simulink model "Fuzzy_PID"  (R2022b)
settings: Solver=FixedStepAuto  StartTime=0.0  StopTime=0.1  FixedStep=0.001  RelTol=1e-3
libraries: fuzblock x1
settings Model: Creator=zhouwenjie  LastModifiedBy=zhouwenjie

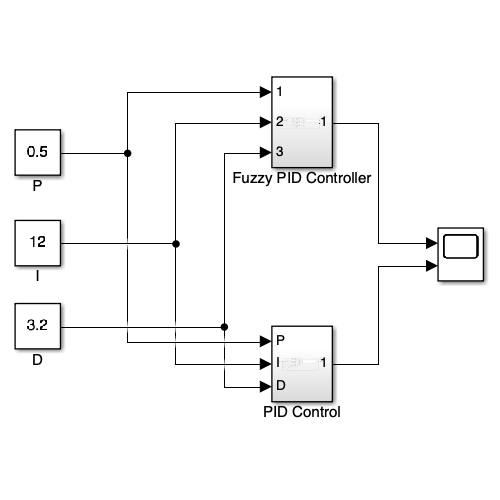
[thumbnail: Simulink's stored preview of the top-level diagram]
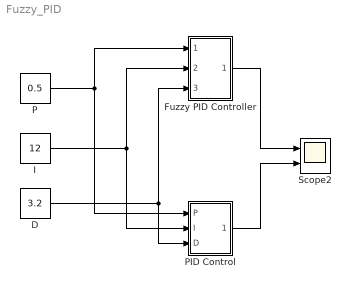
== system Fuzzy_PID ==
  D : Constant  Value=3.2
  Fuzzy PID Controller : Subsystem
  I : Constant  Value=12
  P : Constant  Value=0.5
  PID Control : Subsystem
  Scope2 : Scope  NumInputPorts=2
  wires:
  P/1 -> PID Control/1(P), Fuzzy PID Controller/1(In1)
  I/1 -> PID Control/2(I), Fuzzy PID Controller/2(In2)
  D/1 -> Fuzzy PID Controller/3(In3), PID Control/3(D)
  PID Control/1(Output) -> Scope2/2
  Fuzzy PID Controller/1(Out1) -> Scope2/1

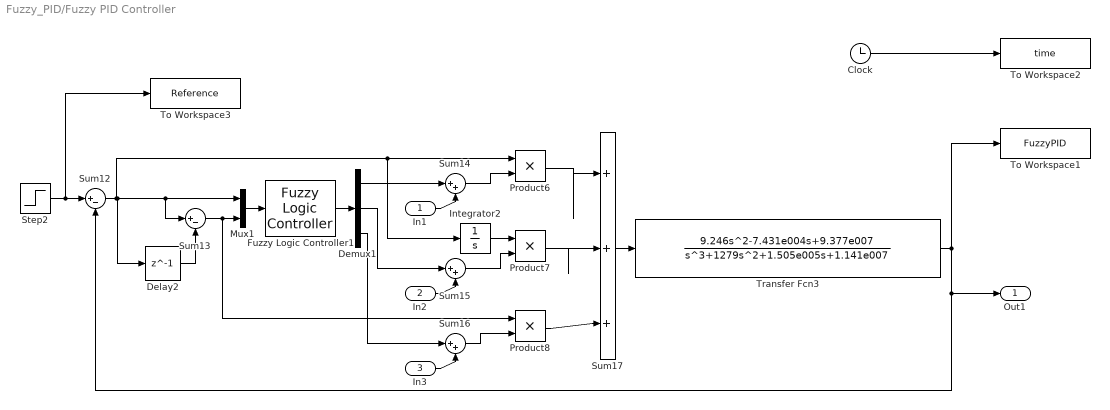
== system Fuzzy_PID/Fuzzy PID Controller ==
  In1 : Inport
  In2 : Inport  Port=2
  In3 : Inport  Port=3
  Clock : Clock
  Delay2 : Delay  DelayLength=1  InitialCondition=1
  Demux1 : Demux  Outputs=3
  Fuzzy Logic Controller1 : fuzblock/Fuzzy Logic  Controller  FIS="\"fuzzy_model\""  OutputSampleNumber=101  DataType=double  FuzzifiedInputs=off  RuleFiringStrengths=off  RuleOutputs=off  AggregatedOutputs=off  SimulateUsing=Interpreted execution  OutOfRangeInputValueMessage=warning  NoRuleFiredMessage=warning  EmptyOutputFuzzySetMessage=warning
  Integrator2 : Integrator
  Mux1 : Mux  Inputs=2
  Product6 : Product
  Product7 : Product
  Product8 : Product
  Step2 : Step  Time=0  SampleTime=1
  Sum12 : Sum  Inputs=|+-
  Sum13 : Sum  Inputs=|+-
  Sum14 : Sum  Inputs=|++
  Sum15 : Sum  Inputs=|++
  Sum16 : Sum  Inputs=|++
  Sum17 : Sum  Inputs=|+++
  To Workspace1 : ToWorkspace  VariableName=FuzzyPID  SaveFormat=Timeseries  SampleTime=-1
  To Workspace2 : ToWorkspace  VariableName=time  SaveFormat=Timeseries  SampleTime=-1
  To Workspace3 : ToWorkspace  VariableName=Reference  SaveFormat=Structure With Time  SampleTime=-1
  Transfer Fcn3 : TransferFcn  Numerator=[9.246,-7.431e004, 9.377e007]  Denominator=[1 ,1279, 1.505e005, 1.141e007]
  Out1 : Outport
  wires:
  Product6/1 -> Sum17/1
  Fuzzy Logic Controller1/1 -> Demux1/1
  Demux1/3 -> Sum16/1
  Mux1/1 -> Fuzzy Logic Controller1/1
  Product7/1 -> Sum17/2
  Sum17/1 -> Transfer Fcn3/1
  In3/1 -> Sum16/2
  In1/1 -> Sum14/2
  Integrator2/1 -> Product7/1
  Sum13/1 -> Product8/1, Mux1/2
  Product8/1 -> Sum17/3
  Transfer Fcn3/1 -> To Workspace1/1, Out1/1, Sum12/2
  Sum12/1 -> Integrator2/1, Product6/1, Delay2/1, Sum13/1, Mux1/1
  In2/1 -> Sum15/2
  Sum14/1 -> Product6/2
  Demux1/2 -> Sum15/1
  Step2/1 -> To Workspace3/1, Sum12/1
  Sum15/1 -> Product7/2
  Sum16/1 -> Product8/2
  Demux1/1 -> Sum14/1
  Delay2/1 -> Sum13/2
  Clock/1 -> To Workspace2/1

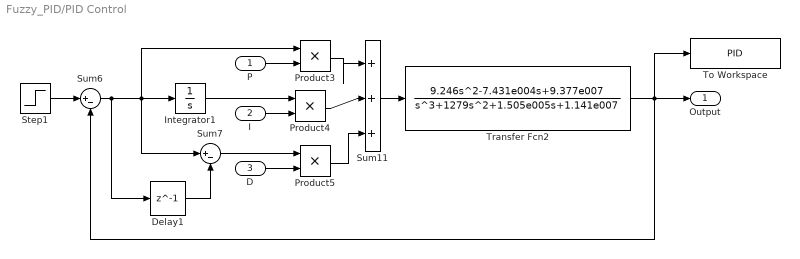
== system Fuzzy_PID/PID Control ==
  P : Inport
  I : Inport  Port=2
  D : Inport  Port=3
  Delay1 : Delay  DelayLength=1  InitialCondition=1
  Integrator1 : Integrator
  Product3 : Product
  Product4 : Product
  Product5 : Product
  Step1 : Step  Time=0  SampleTime=1
  Sum11 : Sum  Inputs=|+++
  Sum6 : Sum  Inputs=|+-
  Sum7 : Sum  Inputs=|+-
  To Workspace : ToWorkspace  VariableName=PID  SaveFormat=Timeseries  SampleTime=-1
  Transfer Fcn2 : TransferFcn  Numerator=[9.246,-7.431e004, 9.377e007]  Denominator=[1 ,1279, 1.505e005, 1.141e007]
  Output : Outport
  wires:
  Step1/1 -> Sum6/1
  Sum6/1 -> Delay1/1, Product3/1, Sum7/1, Integrator1/1
  Delay1/1 -> Sum7/2
  P/1 -> Product3/2
  Integrator1/1 -> Product4/1
  Product5/1 -> Sum11/3
  Sum7/1 -> Product5/1
  Product3/1 -> Sum11/1
  Product4/1 -> Sum11/2
  Transfer Fcn2/1 -> To Workspace/1, Sum6/2, Output/1
  Sum11/1 -> Transfer Fcn2/1
  I/1 -> Product4/2
  D/1 -> Product5/2
